simulink model "pendulumsim"  (Simulink 7.8)
settings: Solver=ode45  StartTime=0.0  StopTime=40  RelTol=1e-3
undefined symbols (not defined in the file or in its folder): controller, drawPendulum, P
settings Model: Creator=Administrator  LastModifiedBy=ecestudent
settings DebuggingCC: FcnCallInpInsideContextMsg=Use local settings  StrictBusMsg=Warning

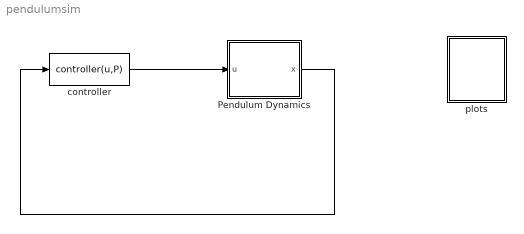
== system pendulumsim ==
  Pendulum Dynamics : Subsystem
      mask Display: image(imread('pend.jpg'))
  controller : MATLABFcn  MATLABFcn=controller(u,P)  OutputDimensions=1  SampleTime=P.Ts
  plots : Subsystem
      mask Display: image(imread('tv.jpg'))
  wires:
  controller/1 -> Pendulum Dynamics/1(u)
  Pendulum Dynamics/1(x) -> controller/1

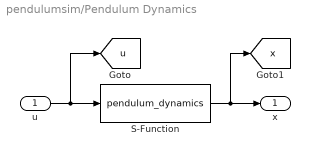
== system pendulumsim/Pendulum Dynamics ==
  u : Inport
  S-Function : S-Function  FunctionName=pendulum_dynamics  Parameters=P  EnableBusSupport=off
  x : Outport
  tag scope: u=global, x=global
  wires:
  u/1 -> S-Function/1, [u]
  S-Function/1 -> x/1, [x]

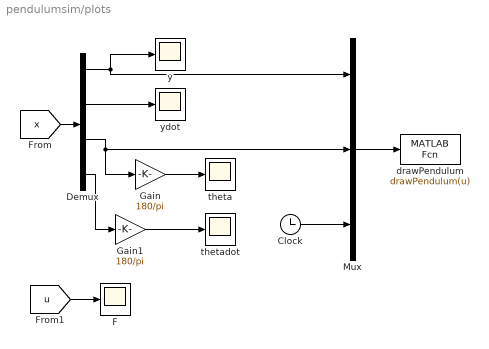
== system pendulumsim/plots ==
  Clock : Clock
  Demux : Demux
  F : Scope
      settings: TimeRange=40  YMin=-10  YMax=15  SaveName=ScopeData4
  Gain : Gain  Gain=180/pi
  Gain1 : Gain  Gain=180/pi
  Mux : Mux  Inputs=3
  drawPendulum : MATLABFcn  MATLABFcn=drawPendulum(u)  OutputDimensions=0  SampleTime=0.1
  theta : Scope
      settings: TimeRange=40  YMin=-2  YMax=1  SaveName=ScopeData2
  thetadot : Scope
      settings: TimeRange=40  YMin=-2  YMax=1  SaveName=ScopeData3
  y : Scope
      settings: TimeRange=40  YMin=-1
  ydot : Scope
      settings: TimeRange=40  YMin=-1  YMax=0.4000000000000001
  wires:
  Demux/1 -> y/1, Mux/1
  Demux/2 -> ydot/1
  [x] -> Demux/1
  Gain/1 -> theta/1
  Demux/3 -> Gain/1, Mux/2
  Gain1/1 -> thetadot/1
  Demux/4 -> Gain1/1
  Mux/1 -> drawPendulum/1
  Clock/1 -> Mux/3
  [u] -> F/1
